simulink model "DACPCScope"  (R2020a)
settings: Solver=FixedStepDiscrete  StartTime=0.0  StopTime=10.0  RelTol=1e-3
undefined symbols (not defined in the file): serial
libraries: instrumentlib x2
settings Model: Creator=oh  LastModifiedBy=oh
settings DataIOCC: ReturnWorkspaceOutputs=off
settings DebuggingCC: ArithmeticOperatorsInVariantConditions=warning
settings SFSimCC: SimUseLocalCustomCode=off  CustomCodeUndefinedFunction=UseInterfaceOnly
settings RTWCC: RTWUseLocalCustomCode=off
settings CodeAppCC: StateflowObjectComments=on

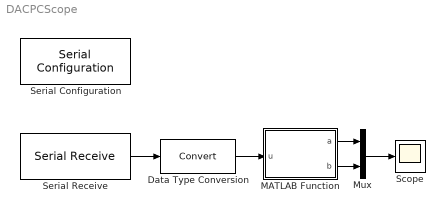
== system DACPCScope ==
  Data Type Conversion : DataTypeConversion
  MATLAB Function : MATLAB Function  TreatAsAtomicUnit=on
  Mux : Mux  Inputs=2
  Scope : Scope
  Serial Configuration : instrumentlib/Serial Configuration  Priority=-200000  ComPortMenu=<Please select a port...>  ComPort=COM3  ObjConstructor=serial('COM3');  BaudRate=115200  DataBits=8  Parity=none  StopBits=1  FlowControl=none  Timeout=10  ByteOrder=LittleEndian
  Serial Receive : instrumentlib/Serial Receive  ComPortMenu=<Please select a port...>  ComPort=COM3  ObjConstructor=serial('COM3');  Terminator=<none>  DataSize=[1 1]  DataType=uint8  EnableBlockingMode=on  ActionDataUnavailable=Output last received value  CustomValue=0  SampleTime=0.001
  wires:
  Serial Receive/1 -> Data Type Conversion/1
  Data Type Conversion/1 -> MATLAB Function/1(u)
  MATLAB Function/1(a) -> Mux/1
  MATLAB Function/2(b) -> Mux/2
  Mux/1 -> Scope/1

== matlab function DACPCScope/MATLAB Function ==
  data: u input; a output; b output
function [a,b]=fcn(u)
coder.extrinsic('sscanf');
persistent array;
persistent idx;
persistent a_old;
persistent b_old;


if isempty(idx)
    idx=1;
end
if isempty(a_old)
    a_old=1.0;
end
if isempty(b_old)
    b_old=1.0;
end
if isempty(array)
    array=zeros(1,50);
end
if  u ~= 10 && u ~= 13
    array(idx) = u;
    idx=idx+1;
end
if u == 13 || idx==50
    disp(char(array));
    disp(size(array));
    c=sscanf(char(array),'%f,%f');
    a_old=c(1);
    b_old=c(2);
    idx=1;
end
a=a_old;
b=b_old;
